simulink model "engs147_ski_jump_motor_model"  (R2024b)
settings: Solver=VariableStepAuto  StartTime=0.0  StopTime=10.0  RelTol=1e-3
model workspace (MAT data in the model file):
  R_a = 0.0951
values from neighbouring files (symbols this model uses):
  gear_ratio = 12    [engs147_body_char.m]    (also in engs147_ski_jump_motor.m; engs147_step_body.m; engs147_wheel_modelling.m)
  J_car = I_car    (= 0.00021786984624)    [engs147_body_char.m]    (also in engs147_ski_jump_motor.m; engs147_step_body.m; engs147_wheel_modelling.m)
  J_rotor = 6.00276e-5    (= 6.00276e-05)    [engs147_body_char.m]    (also in engs147_ski_jump_motor.m; engs147_step_body.m; engs147_wheel_modelling.m = 2.37825655651e-05)
  K_b = 0.00604325    [engs147_body_char.m]    (also in engs147_ski_jump_motor.m; engs147_step_body.m; engs147_wheel_modelling.m = 0.00545154895462)
  K_torque = 0.01    [engs147_body_char.m]    (also in engs147_ski_jump_motor.m; engs147_step_body.m; engs147_wheel_modelling.m)
libraries: simulink x1
settings Model: Creator=noahd  LastModifiedBy=noahd

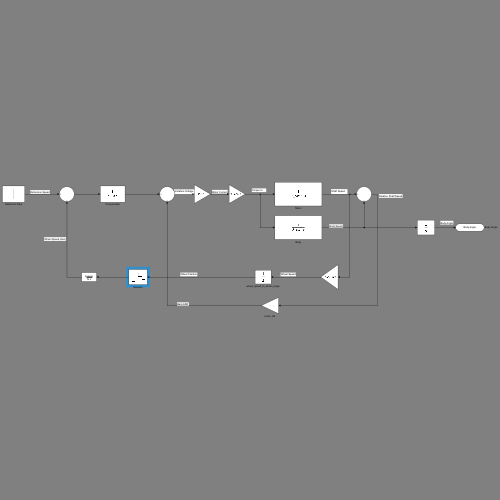
[thumbnail: Simulink's stored preview of the top-level diagram]
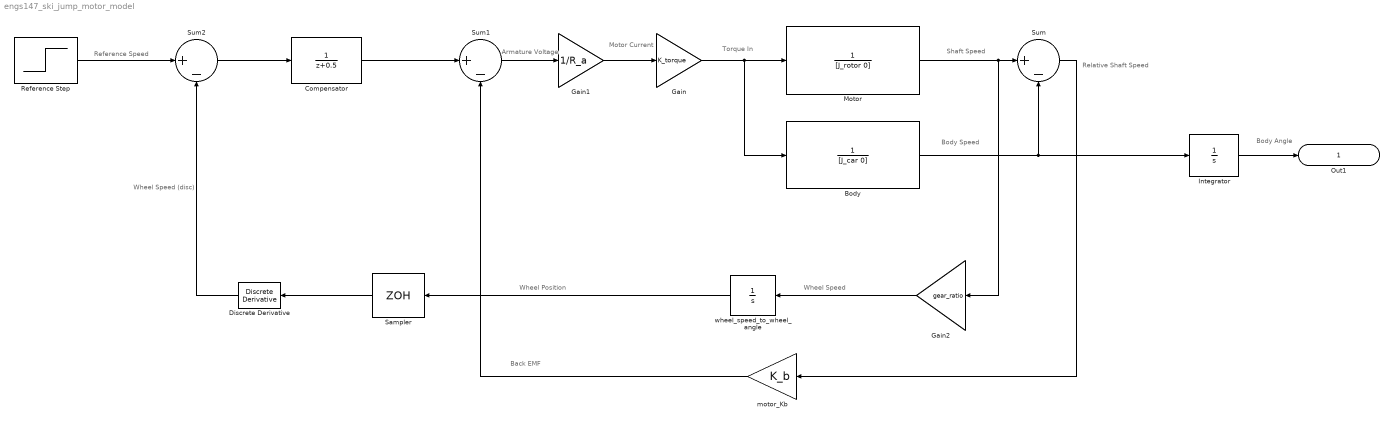
== system engs147_ski_jump_motor_model ==
  note: Reference Speed
  note: Wheel Speed (disc)
  note: Relative Shaft Speed
  note: Back EMF
  note: Wheel Position
  note: Wheel Speed
  note: Body Angle
  note: Body Speed
  note: Armature Voltage
  note: Motor Current
  note: Torque In
  note: Shaft Speed
  Body : TransferFcn  Denominator=[J_car 0]
  Compensator : DiscreteTransferFcn
  Discrete Derivative : simulink/Discrete/Discrete Derivative  gainval=1.0  ICPrevScaledInput=0.0  OutMin=[]  OutMax=[]  OutDataType=fixdt(1, 16)  OutScaling=2^-10  DoSatur=off
  Gain : Gain  Gain=K_torque
  Gain1 : Gain  Gain=1/R_a
  Gain2 : Gain  Gain=gear_ratio
  Integrator : Integrator
  Motor : TransferFcn  Denominator=[J_rotor 0]
  Reference Step : Step  SampleTime=0
  Sampler : ZeroOrderHold  SampleTime=-1
  Sum : Sum  Inputs=|+-
  Sum1 : Sum  Inputs=|+-
  Sum2 : Sum  Inputs=|+-
  motor_Kb : Gain  Gain=K_b
  wheel_speed_to_wheel_angle : Integrator
  Out1 : Outport  SignalName=Body Angle
  wires:
  Gain/1 -> Body/1, Motor/1
  Gain1/1 -> Gain/1
  Body/1 -> Integrator/1, Sum/2
  Motor/1 -> Sum/1, Gain2/1
  Gain2/1 -> wheel_speed_to_wheel_angle/1
  Sum/1 -> motor_Kb/1
  motor_Kb/1 -> Sum1/2
  Sum1/1 -> Gain1/1
  Discrete Derivative/1 -> Sum2/2
  Reference Step/1 -> Sum2/1
  Sum2/1 -> Compensator/1
  Sampler/1 -> Discrete Derivative/1
  wheel_speed_to_wheel_angle/1 -> Sampler/1
  Compensator/1 -> Sum1/1
  Integrator/1 -> Out1/1
